simulink model "control"  (R2021b)
settings: Solver=VariableStepAuto  StartTime=0.0  StopTime=10.0  RelTol=1e-3
settings Model: Creator=hukai  LastModifiedBy=hukai

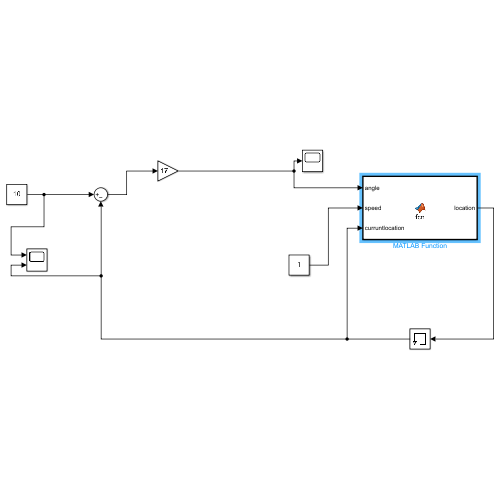
[thumbnail: Simulink's stored preview of the top-level diagram]
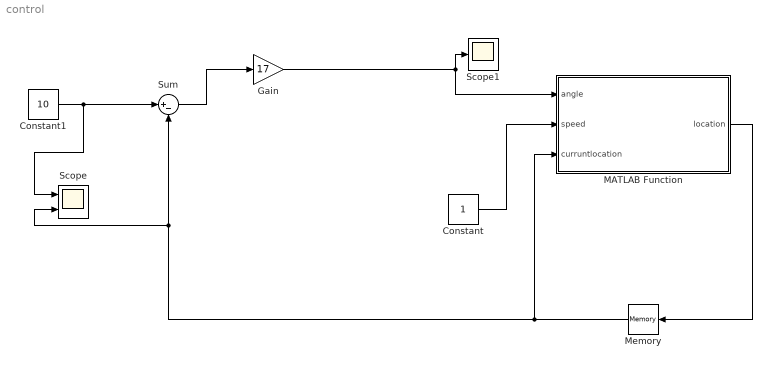
== system control ==
  Constant : Constant
  Constant1 : Constant  Value=10
  Gain : Gain  Gain=17
  MATLAB Function : MATLAB Function  TreatAsAtomicUnit=on
  Memory : Memory  InitialCondition=20
  Scope : Scope  NumInputPorts=2
  Scope1 : Scope
  Sum : Sum  Inputs=|+-
  wires:
  MATLAB Function/1(location) -> Memory/1
  Memory/1 -> MATLAB Function/3(curruntlocation), Scope/2, Sum/2
  Constant/1 -> MATLAB Function/2(speed)
  Constant1/1 -> Scope/1, Sum/1
  Sum/1 -> Gain/1
  Gain/1 -> MATLAB Function/1(angle), Scope1/1

== matlab function control/MATLAB Function ==
  data: angle input; location output; speed input; curruntlocation input
function location = fcn(angle,speed,curruntlocation)
angle = angle/360*2*pi
location = curruntlocation+speed*sin(angle)
